simulink model "p"  (Simulink 2.09)
settings: Solver=ode45  StartTime=0.0  StopTime=260  RelTol=1e-3  AbsTol=1e-3
settings Model: SaveTime=off  SaveOutput=off  ConsistencyChecking=off  RTWTemplateMakefile=grt_vc.tmf

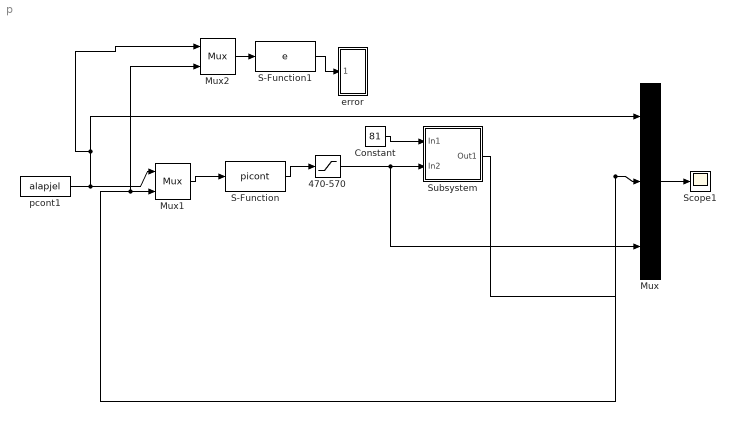
== system p ==
  470-570 : Saturate  UpperLimit=570  LowerLimit=470
  Constant : Constant  Value=81
  Mux : Mux  Inputs=3
  Mux1 : Mux  Inputs=2
  Mux2 : Mux  Inputs=2
  S-Function : S-Function  FunctionName=picont
  S-Function1 : S-Function  FunctionName=e
  Scope1 : Scope
      settings: TickLabels=on  TimeRange=260  YMin=6  YMax=12  SaveName=ki  SampleInput=on
  Subsystem : Subsystem
  error : Subsystem
      mask Display: disp('IAE')
  pcont1 : S-Function  FunctionName=alapjel
  wires:
  Mux/1 -> Scope1/1
  470-570/1 -> Mux/3, Subsystem/2(In2)
  Constant/1 -> Subsystem/1(In1)
  Mux2/1 -> S-Function1/1
  S-Function1/1 -> error/1(in_1)
  S-Function/1 -> 470-570/1
  pcont1/1 -> Mux2/1, Mux/1, Mux1/1
  Mux1/1 -> S-Function/1
  Subsystem/1(Out1) -> Mux2/2, Mux1/2, Mux/2

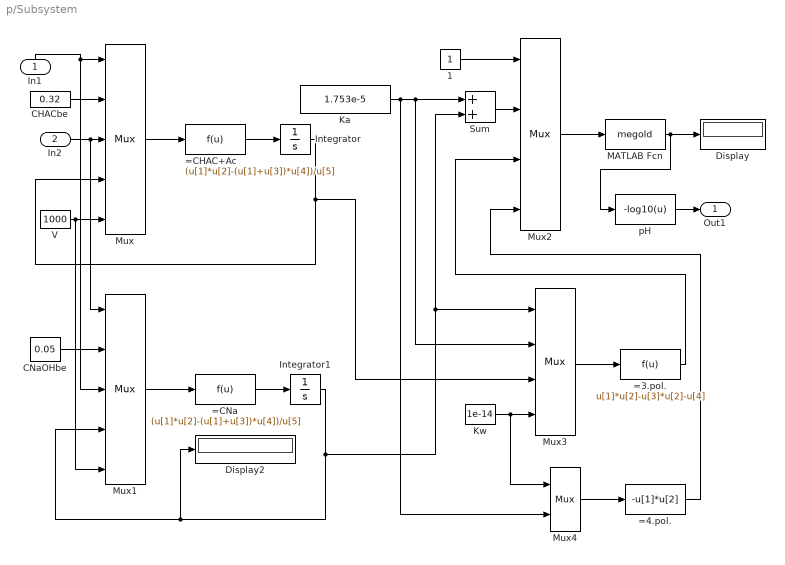
== system p/Subsystem ==
  In1 : Inport  Orientation=up  Port=1  PortWidth=-1  SampleTime=-1
  In2 : Inport  Port=2  PortWidth=-1  SampleTime=-1
  1 : Constant  Value=1
  =3.pol. : Fcn  Expr=u[1]*u[2]-u[3]*u[2]-u[4]
  =4.pol. : Fcn  Expr=-u[1]*u[2]
  =CHAC+Ac : Fcn  Expr=(u[1]*u[2]-(u[1]+u[3])*u[4])/u[5]
  =CNa : Fcn  Expr=(u[1]*u[2]-(u[1]+u[3])*u[4])/u[5]
  CHACbe : Constant  Value=0.32
  CNaOHbe : Constant  Value=0.05
  Display : Display
      settings: Format=short
  Display2 : Display
      settings: Format=short
  Integrator : Integrator  ExternalReset=none  InitialConditionSource=internal  InitialCondition=0.0435  LimitOutput=off  UpperSaturationLimit=inf  LowerSaturationLimit=-inf  ShowSaturationPort=off  ShowStatePort=off  AbsoluteTolerance=auto
  Integrator1 : Integrator  ExternalReset=none  InitialConditionSource=internal  InitialCondition=0.0432  LimitOutput=off  UpperSaturationLimit=inf  LowerSaturationLimit=-inf  ShowSaturationPort=off  ShowStatePort=off  AbsoluteTolerance=auto
  Ka : Constant  Value=1.753e-5
  Kw : Constant  Value=1e-14
  MATLAB Fcn : MATLABFcn  MATLABFcn=megold  OutputWidth=1
  Mux : Mux  Inputs=5
  Mux1 : Mux  Inputs=5
  Mux2 : Mux  Inputs=4
  Mux3 : Mux  Inputs=4
  Mux4 : Mux  Inputs=2
  Sum : Sum  Inputs=++
  V : Constant  Value=1000
  pH : Fcn  Expr=-log10(u)
  Out1 : Outport  Port=1  InitialOutput=0
  wires:
  pH/1 -> Out1/1
  MATLAB Fcn/1 -> pH/1, Display/1
  Mux2/1 -> MATLAB Fcn/1
  =4.pol./1 -> Mux2/4
  =3.pol./1 -> Mux2/3
  Sum/1 -> Mux2/2
  Ka/1 -> Mux4/2, Mux3/2, Sum/1
  Kw/1 -> Mux4/1, Mux3/4
  Mux4/1 -> =4.pol./1
  Integrator/1 -> Mux3/3, Mux/4
  Mux3/1 -> =3.pol./1
  Integrator1/1 -> Mux3/1, Sum/2, Mux1/4, Display2/1
  1/1 -> Mux2/1
  V/1 -> Mux1/5, Mux/5
  Mux1/1 -> =CNa/1
  =CNa/1 -> Integrator1/1
  In1/1 -> Mux1/3, Mux/1
  CNaOHbe/1 -> Mux1/2
  In2/1 -> Mux1/1, Mux/3
  =CHAC+Ac/1 -> Integrator/1
  Mux/1 -> =CHAC+Ac/1
  CHACbe/1 -> Mux/2

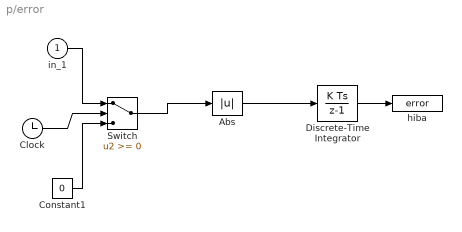
== system p/error ==
  in_1 : Inport  Port=1  PortWidth=-1  SampleTime=-1
  Abs : Abs
  Clock : Clock
  Constant1 : Constant  Value=0
  Discrete-Time Integrator : DiscreteIntegrator  IntegratorMethod=ForwardEuler  ExternalReset=none  InitialConditionSource=internal  InitialCondition=0  LimitOutput=off  UpperSaturationLimit=inf  LowerSaturationLimit=-inf  ShowSaturationPort=off  ShowStatePort=off  SampleTime=0.2
  Switch : Switch  Threshold=0
  hiba : ToWorkspace  VariableName=error  SampleTime=0
      settings: Buffer=1
  wires:
  Switch/1 -> Abs/1
  in_1/1 -> Switch/1
  Constant1/1 -> Switch/3
  Clock/1 -> Switch/2
  Abs/1 -> Discrete-Time Integrator/1
  Discrete-Time Integrator/1 -> hiba/1
